simulink model "rtwdemo_configwizard"  (Simulink 7.6)
settings: Solver=FixedStepDiscrete  StartTime=0.0  StopTime=48  FixedStep=1  RelTol=1e-3  SampleTimeConstraint=STIndependent
PostLoadFcn:
  | INC=uint8(1);LIMIT=uint8(16);RESET=uint8(0);K=int32(2);
Description:
  | Configuring a Model for Code Generation
settings Model: Creator=The MathWorks Inc.  ParamWorkspaceSource=ReferencedWorkspace  CovMetricSettings=d  ExtModeTrigMode=oneshot  ExtModeArmWhenConnect=off  ExtModeAutoUpdateStatusClock=off
settings MATStruct: SampleTime=1  Offset=0  Priority=[41.0]
settings DataIOCC: LimitDataPoints=off  SaveFormat=StructureWithTime  SaveOutput=off  SaveTime=off  SignalLoggingName=sigsOut
settings OptimizationCC: InlineParams=on  InlineInvariantSignals=on  StateBitsets=on  DataBitsets=on  UseTempVars=on  EfficientFloat2IntCast=on  EfficientMapNaN2IntZero=off  BufferReusableBoundary=off
settings DebuggingCC: CheckExecutionContextPreStartOutputMsg=on  CheckExecutionContextRuntimeOutputMsg=on  SolverPrmCheckMsg=none  IntegerOverflowMsg=none  StrictBusMsg=ErrorOnBusTreatedAsVector
settings HardwareCC: ProdIntDivRoundTo=Zero  ProdEndianess=LittleEndian  ProdHWDeviceType=Generic->32-bit Embedded Processor  TargetHWDeviceType=Generic->32-bit Embedded Processor
settings ModelReferenceCC: UpdateModelReferenceTargets=IfOutOfDate
settings RTWCC: TLCOptions=-p0  GenCodeOnly=on  GenerateReport=on  RTWVerbose=off  ProcessScript=grt_make_rtw_hook  LaunchReport=on  GenerateCodeInfo=on
settings CodeAppCC: ForceParamTrailComments=on

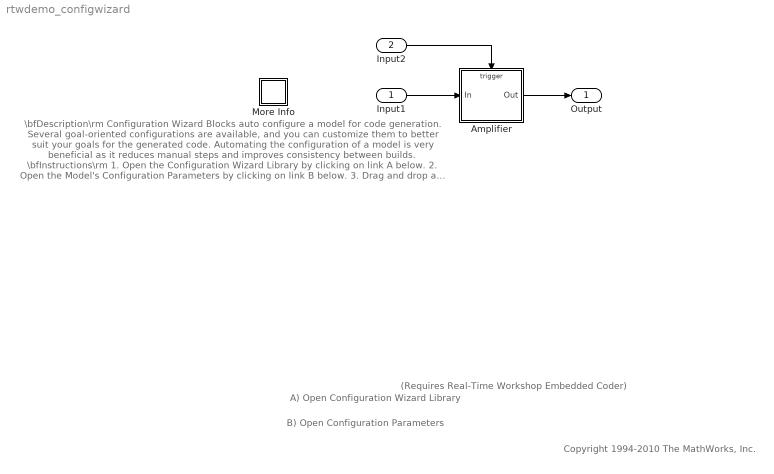
== system rtwdemo_configwizard ==
  note: \bfDescription\rm
      | Configuration Wizard Blocks auto configure a model for code generation.  Several
      | goal-oriented configurations are available, and you can customize them to better suit
      | your goals for the generated code.  Automating the configuration of a model is very
      | beneficial as it reduces manual steps and improves consistency between builds.
      |
      | \bfInstructions\rm
      | 1. Open the Configuration Wizard Library by clicking on link A below.
      | 2. Open the Model's Configuration Parameters by clicking on link B below.
      | 3. Drag and drop a Configuration Wizard Block, for example ERT (optimized for fixed-
      |     point), from the wizard library into the model.
      | 4. Double-click the wizard block.
      | 5. Note that the Configuration Parameter options are modified automatically.
  note: Copyright 1994-2010 The MathWorks, Inc.
  note: A) Open Configuration Wizard Library
  note: B) Open Configuration Parameters
  note: (Requires Real-Time Workshop Embedded Coder)
  Input1 : Inport  OutDataTypeStr=int32  PortDimensions=1
  Input2 : Inport  Port=2  OutDataTypeStr=int32  PortDimensions=1
  Amplifier : Subsystem  TreatAsAtomicUnit=on
  More Info : Subsystem
      settings: OpenFcn=showdemo('rtwdemo_configuration_set')
      mask Display: disp('?')
  Output : Outport
  wires:
  Input1/1 -> Amplifier/1(In)
  Amplifier/1(Out) -> Output/1
  Input2/1 -> Amplifier/Trigger

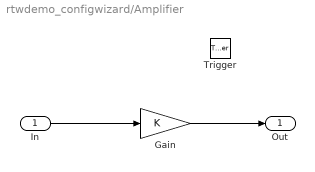
== system rtwdemo_configwizard/Amplifier ==
  In : Inport
  Trigger : TriggerPort
  Gain : Gain  Gain=K  OutDataTypeStr=Inherit: Same as input  ParamDataTypeStr=Inherit: Same as input
  Out : Outport  InitialOutput=0
  wires:
  In/1 -> Gain/1
  Gain/1 -> Out/1

== system rtwdemo_configwizard/More Info ==
